simulink model "SmartMeter"  (R2023b)
settings: Solver=VariableStepAuto  StartTime=0.0  StopTime=3600*7.5  RelTol=1e-3
InitFcn:
  | Ts = 1; % Step time as 1second
StopFcn:
  | plotResults = true ;% turn off if unwanted
  | 
  | if plotResults
  | 
  | out = out_SmartMeterModel.SmartMeterValidationScope;
  | 
  | % Get Signals from simulation output.
  | time = out.time;
  | TestSignal = out.signals.values(:,1);
  | E_meas_15min = out.signals.values(:,2:3);
  | E_meas_hourly = out.signals.values(:,4:5);
  | price = out.signals.values(:,6:7);
  | Bill_hourly = out.signals.values(:,8:9);
  | 
  | %% Create Figure
  | fig_SmartMeterValidation_Results = figure;
  | 
  | % X-axis
  | step = 3600;
  | myxtick = 0:step:time(end);
  | myxticklabel = 0:time(end)/step ;
  | 
  | % TestSignal
  | subplot(5,1,1);
  | hold on;
  | plot(time, TestSignal, '-', 'LineWidth', 2,'Color','black');
  | ylim 'padded'
  | ylabel('Power (kW)');
  | xticks(myxtick);
  | xticklabels(myxticklabel);
  | xlim 'tight'
  | xlabel('Time (hours)');
  | title('Power');
  | grid on;
  | box on
  | 
  | % E 15
  | subplot(5,1,2);
  | hold on
  | stairs(time, E_meas_15min(:,1), 'LineWidth', 2);
  | stairs(time, E_meas_15min(:,2), 'LineWidth', 2);
  | ylim 'padded'
  | yticks(-1:0.25:1)
  | ylabel('Energy (kWh)');
  | xticks(myxtick);
  | xticklabels(myxticklabel);
  | xlim 'tight'
  | xlabel('Time (hours)');
  | %legend('BattPower','Location', 'northwest')
  | title('Measurements 15 min interval');
  | grid on;
  | box on
  | 
  | % E hourly
  | subplot(5,1,3);
  | hold on
  | stairs(time, E_meas_hourly(:,1), 'LineWidth', 2);
  | stairs(time, E_meas_hourly(:,2), 'LineWidth', 2);
  | ylim 'padded'
  | yticks(0:0.5:2)
  | ylabel('Energy (kWh)');
  | xticks(myxtick);
  | xticklabels(myxticklabel);
  | xlabel('Time (hours)');
  | xlim 'tight'
  | %legend('BattPower','Location', 'northwest')
  | title('Measurements hourly');
  | grid on;
  | box on
  | 
  | % price
  | subplot(5,1,4);
  | hold on
  | plot(time, price(:,1),':', 'LineWidth', 2,'Color','black')
  | plot(time, price(:,2),'-', 'LineWidth', 2,'Color','black')
  | ylim 'padded'
  | ylabel('DKK per kWh','Color','black');
  | xticks(myxtick);
  | xticklabels(myxticklabel);
  | xlim 'tight'
  | xlabel('Time (hours)');
  | legend( 'price','price shifted','Location', 'northeast');%, 'Location', 'northeast', 'Orientation', 'vertical', 'Position', [0.75, 0.2, 0.05, 0.05]);
  | title('Electricity spot price');
  | grid on;
  | box on
  | 
  | 
  | % Bill_hourly
  | subplot(5,1,5);
  | hold on
  | plot(time, Bill_hourly(:,1),'-', 'LineWidth', 2)
  | plot(time, Bill_hourly(:,2),'-', 'LineWidth', 2)
  | ylim 'padded'
  | ylabel('DKK');
  | xlim 'tight'
  | xticks(myxtick);
  | xticklabels(myxticklabel);
  | xlabel('Time (hours)');
  | %legend( 'price','price shifted','Location', 'northeast');
  | title('Hourly bill');
  | grid on;
  | box on
  | 
  | % Stretch Figure
  | figwidth = 8; % Width in inches
  | figheight = 6; % Height in inches
  | set(gcf, 'Units', 'Inches', 'Position', [1, 1, figwidth, figheight]);
  | 
  | % Save Files
  | saveas(fig_SmartMeterValidation_Results, 'SmartMeterValidation_Results', 'epsc')
  | saveas(fig_SmartMeterValidation_Results, 'SmartMeterValidation_Results', 'pdf')
  | 
  | disp('Figures saved as PDF and eps')
  | 
  | 
  | 
  | 
  | 
  | end
undefined symbols (not defined in the file): DiscIntNeverNeededParam, sigbuilder_block
libraries: dspsigops x2, spspowerguiLib x1
settings Model: Creator=leons  LastModifiedBy=leons
settings DataIOCC: ReturnWorkspaceOutputsName=out_SmartMeterModel

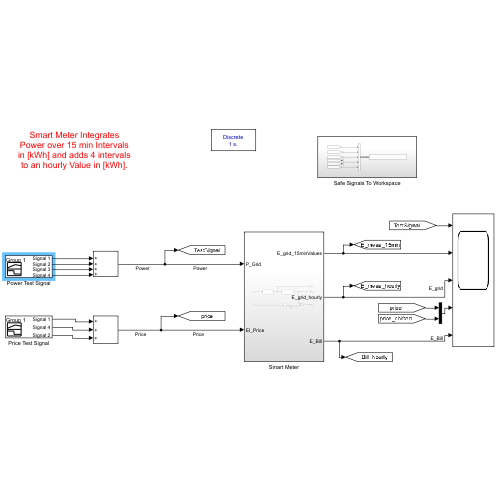
[thumbnail: Simulink's stored preview of the top-level diagram]
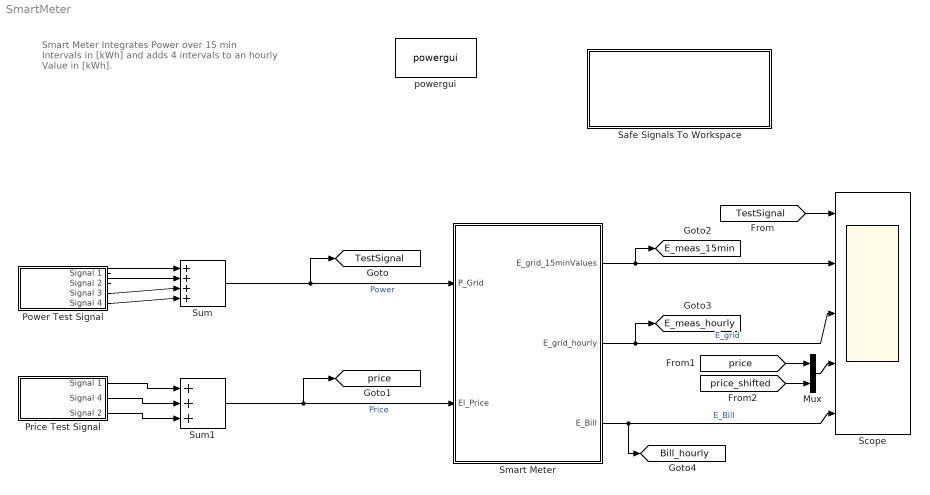
== system SmartMeter ==
  note: Smart Meter Integrates Power over 15 min Intervals in [kWh] and adds 4 intervals to an hourly Value in [kWh].
  Mux : Mux  Inputs=2
  Power Test Signal : Subsystem  Tag=STV Subsys  LoadFcn=sigbuilder_block('load');  StartFcn=sigbuilder_block('start');  StopFcn=sigbuilder_block('stop');  ClipboardFcn=sigbuilder_block('clipboard');  mask(Sigbuilder block){tuvar=[0:10]}
      mask help: Simulink:masks:SigbuilderBlock_MD
      mask init:
      | if ~strcmp(get_param(bdroot(gcbh),'SimulationStatus'),'stopped') tuvar = sigbuilder_block('maskInit'); end
      settings: CopyFcn=sigbuilder_block('copy');  DeleteFcn=sigbuilder_block('delete');  ModelCloseFcn=sigbuilder_block('modelClose');  PreSaveFcn=sigbuilder_block('preSave');  PauseFcn=sigbuilder_block('pause');  ContinueFcn=sigbuilder_block('continue');  NameChangeFcn=sigbuilder_block('namechange');  OpenFcn=sigbuilder_block('open',[38.4 99 759.6 460.8 ]);  CloseFcn=sigbuilder_block('close');
      mask Display: plot(0, 0, 100, 100,[2, 2, 32, 32, 2], [68, 8, 8, 68, 68],[32, 2], [38, 38], [32, 19, 2],[53, 60, 44], [32, 17, 17, 2],[16, 16, 31, 31]);txt = getActiveGroup(gcbh);text(2, 100, txt,'verticalAlignment', 'top');
  Price Test Signal : Subsystem  Tag=STV Subsys  LoadFcn=sigbuilder_block('load');  StartFcn=sigbuilder_block('start');  StopFcn=sigbuilder_block('stop');  ClipboardFcn=sigbuilder_block('clipboard');  mask(Sigbuilder block){tuvar=[0:10]}
      mask help: Simulink:masks:SigbuilderBlock_MD
      mask init:
      | if ~strcmp(get_param(bdroot(gcbh),'SimulationStatus'),'stopped') tuvar = sigbuilder_block('maskInit'); end
      settings: CopyFcn=sigbuilder_block('copy');  DeleteFcn=sigbuilder_block('delete');  ModelCloseFcn=sigbuilder_block('modelClose');  PreSaveFcn=sigbuilder_block('preSave');  PauseFcn=sigbuilder_block('pause');  ContinueFcn=sigbuilder_block('continue');  NameChangeFcn=sigbuilder_block('namechange');  OpenFcn=sigbuilder_block('open',[110.4 45 759.6 460.8 ]);  CloseFcn=sigbuilder_block('close');
      mask Display: plot(0, 0, 100, 100,[2, 2, 32, 32, 2], [68, 8, 8, 68, 68],[32, 2], [38, 38], [32, 19, 2],[53, 60, 44], [32, 17, 17, 2],[16, 16, 31, 31]);txt = getActiveGroup(gcbh);text(2, 100, txt,'verticalAlignment', 'top');
  Safe Signals To Workspace : Subsystem
  Scope : Scope  NumInputPorts=5
  Smart Meter : Subsystem
  Sum : Sum  Inputs=|++++
  Sum1 : Sum  Inputs=+++
  powergui : spspowerguiLib/powergui  Priority=1  SimulationMode=Discrete  SampleTime=Ts  frequency=60  Iterations=50  frequencyindice=60  Pbase=100e6  ErrMax=1e-4  UnitsV=kV  UnitsW=MW  buscounter=0  FunctionMessages=off  echomessages=off  EnableUseOfTLC=off  CurrentSourceSwitches=off  DisableSnubberDevices=off  DisableRonSwitches=off  DisableVfSwitches=off  DisplayEquations=off  AutomaticDiscreteSolvers=off  SolverType=Tustin/Backward Euler (TBE)  Interpol=off  ExternalGateDelay=off  methode=off  Ts=100  x0status=blocks  SPID=on  SwTol=0  HookPort=off  NonlinearTolerance=1e-4  nMaxIteration=100  ContinueOnMaxIteration=off  RestoreLinks=warning  ResistiveCurrentMeasurement=off  Frange=[0:2:500]  Ylog=off  Xlog=on  ShowGrid=off  save=off  variable=ZData  structure=0  ZoomFFT=off  StartTime=0.0  cycles=1  DisplayStyle=1  fundamental=60  FreqAxis=off  MaxFrequency=1000  frequencyindicesteady=1  RmsSteady=1  display=off
  tag scope: Bill_hourly=global, E_meas_15min=global, E_meas_hourly=global, TestSignal=global, price=global
  wires:
  Smart Meter/2(E_grid_hourly) -> [E_meas_hourly], Scope/3  "E_grid"
  Power Test Signal/4(Signal 4) -> Sum/4
  Power Test Signal/2(Signal 2) -> Sum/2
  Power Test Signal/1(Signal 1) -> Sum/1
  Power Test Signal/3(Signal 3) -> Sum/3
  Price Test Signal/1(Signal 1) -> Sum1/1
  Price Test Signal/2(Signal 4) -> Sum1/2
  Sum1/1 -> Smart Meter/2(El_Price), [price]  "Price"
  Smart Meter/3(E_Bill) -> Scope/5, [Bill_hourly]  "E_Bill"
  [TestSignal] -> Scope/1
  [price] -> Mux/1
  Sum/1 -> [TestSignal], Smart Meter/1(P_Grid)  "Power"
  Smart Meter/1(E_grid_15minValues) -> [E_meas_15min], Scope/2
  Mux/1 -> Scope/4
  [price_shifted] -> Mux/2
  Price Test Signal/3(Signal 2) -> Sum1/3

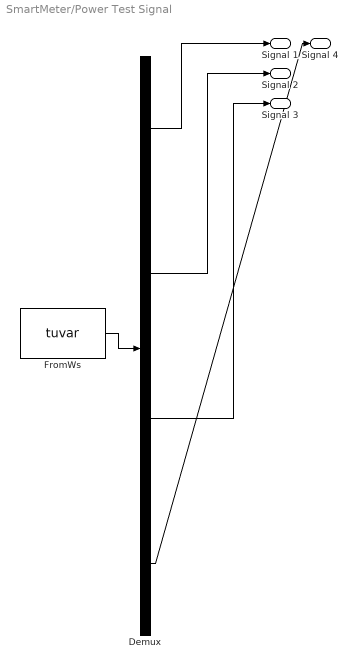
== system SmartMeter/Power Test Signal ==
  Demux : Demux  Tag=STV Demux
      settings: DisplayOption=none
  FromWs : FromWorkspace  Tag=STV FromWs  VariableName=tuvar
      SigBuilderData=|
      | common.afterFinalStr = 'Extrapolate'
      | common.sampleTime = 0
      | dataSet.timeRange = [0 25200]
      | dataSet.name = 'Group 1'
      | sbobj.Groups.Name = 'Group 1'
      | sbobj.Groups.Signals(1).Name = 'Signal 1'
      | sbobj.Groups.Signals(1).XData = [0 1 1 3600 3600 25200]
      | sbobj.Groups.Signals(1).YData = [0 0 1 1 0 0]
      | sbobj.Groups.Signals(2).Name = 'Signal 2'
      | sbobj.Groups.Signals(2).XData = [0 3600 3600 12600 12600 25200]
      | sbobj.Groups.Signals(2).YData = [0 0 2 2 0 0]
      | sbobj.Groups.Signals(3).Name = 'Signal 3'
      | sbobj.Groups.Signals(3).XData = [0 14402 14402 15298 15298 25200]
      | sbobj.Groups.Signals(3).YData = [0 0 2 -2 0 0]
      | sbobj.Groups.Signals(4).Name = 'Signal 4'
      | sbobj.Groups.Signals(4).XData = [0 18000 18000 19800 19800 25200]
      | sbobj.Groups.Signals(4).YData = [0 0 2 -2 0 0]
      | sbobj.Groups.TimeRange = [0 25200]
  Signal 1 : Outport  Tag=STV Outport
  Signal 2 : Outport  Tag=STV Outport  Port=2
  Signal 3 : Outport  Tag=STV Outport  Port=3
  Signal 4 : Outport  Tag=STV Outport  Port=4
  wires:
  Demux/3 -> Signal 3/1
  Demux/2 -> Signal 2/1
  FromWs/1 -> Demux/1
  Demux/1 -> Signal 1/1
  Demux/4 -> Signal 4/1

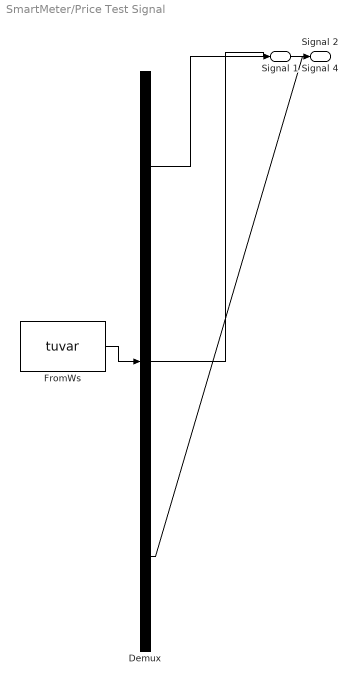
== system SmartMeter/Price Test Signal ==
  Demux : Demux  Tag=STV Demux  Outputs=3
      settings: DisplayOption=none
  FromWs : FromWorkspace  Tag=STV FromWs  VariableName=tuvar
      SigBuilderData=|
      | common.afterFinalStr = 'Extrapolate'
      | common.sampleTime = 0
      | dataSet.timeRange = [0 25200]
      | dataSet.name = 'Group 1'
      | sbobj.Groups.Name = 'Group 1'
      | sbobj.Groups.Signals(1).Name = 'Signal 1'
      | sbobj.Groups.Signals(1).XData = [0 1 1 3600 3600 25200]
      | sbobj.Groups.Signals(1).YData = [0 0 2 2 0 0]
      | sbobj.Groups.Signals(2).Name = 'Signal 4'
      | sbobj.Groups.Signals(2).XData = [0 7200 7200 25200]
      | sbobj.Groups.Signals(2).YData = [0 0 1 1]
      | sbobj.Groups.Signals(3).Name = 'Signal 2'
      | sbobj.Groups.Signals(3).XData = [0 3600 3600 7200 7200 25200]
      | sbobj.Groups.Signals(3).YData = [0 0 3 3 0 0]
      | sbobj.Groups.TimeRange = [0 25200]
  Signal 1 : Outport  Tag=STV Outport
  Signal 4 : Outport  Tag=STV Outport  Port=2
  Signal 2 : Outport  Tag=STV Outport  Port=3
  wires:
  FromWs/1 -> Demux/1
  Demux/1 -> Signal 1/1
  Demux/2 -> Signal 4/1
  Demux/3 -> Signal 2/1

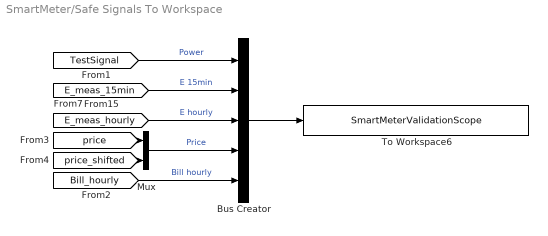
== system SmartMeter/Safe Signals To Workspace ==
  Bus Creator : BusCreator  Inputs=5
  Mux : Mux  Inputs=2
  To Workspace6 : ToWorkspace  VariableName=SmartMeterValidationScope  SaveFormat=Structure With Time  SampleTime=-1
  wires:
  Bus Creator/1 -> To Workspace6/1
  [E_meas_15min] -> Bus Creator/2  "E 15min"
  [TestSignal] -> Bus Creator/1  "Power"
  [E_meas_hourly] -> Bus Creator/3  "E hourly"
  Mux/1 -> Bus Creator/4  "Price"
  [Bill_hourly] -> Bus Creator/5  "Bill hourly"
  [price_shifted] -> Mux/2
  [price] -> Mux/1

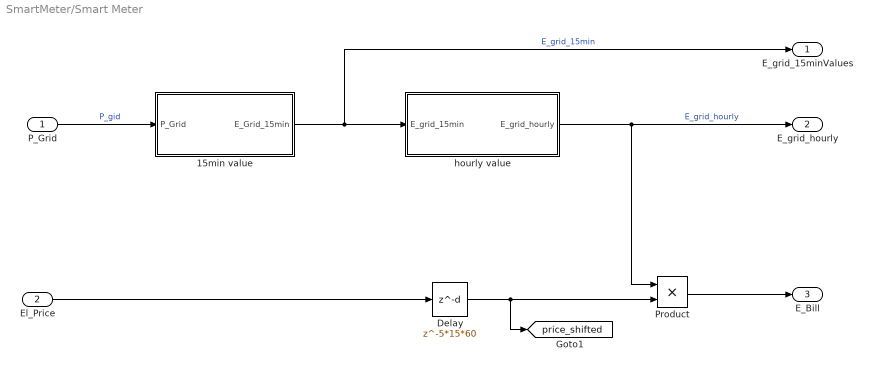
== system SmartMeter/Smart Meter ==
  P_Grid : Inport
  El_Price : Inport  Port=2
  15min value : Subsystem
  Delay : Delay  DelayLength=5*15*60  SampleTime=1
  Product : Product
  hourly value : Subsystem
  E_grid_15minValues : Outport
  E_grid_hourly : Outport  Port=2
  E_Bill : Outport  Port=3
  tag scope: price_shifted=global
  wires:
  P_Grid/1 -> 15min value/1(P_Grid)  "P_gid"
  15min value/1(E_Grid_15min) -> E_grid_15minValues/1, hourly value/1(E_grid_15min)  "E_grid_15min"
  hourly value/1("E_grid_hourly ") -> E_grid_hourly/1, Product/1  "E_grid_hourly"
  El_Price/1 -> Delay/1
  Delay/1 -> [price_shifted], Product/2
  Product/1 -> E_Bill/1

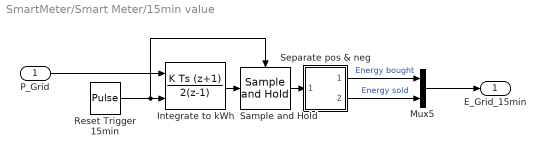
== system SmartMeter/Smart Meter/15min value ==
  P_Grid : Inport
  Integrate to kWh : DiscreteIntegrator  IntegratorMethod=Integration: Trapezoidal  gainval=1/(3600)  ExternalReset=falling  SampleTime=-1  ICPrevOutput=DiscIntNeverNeededParam  ICPrevScaledInput=DiscIntNeverNeededParam
  Mux5 : Mux  Inputs=2
  Reset Trigger 15min : DiscretePulseGenerator  Period=15*60  SampleTime=Ts
  Sample and Hold : dspsigops/Sample and Hold  trig=Rising edge  initCond=0  latchinput=off
  Separate pos & neg : Subsystem
  E_Grid_15min : Outport
  wires:
  Integrate to kWh/1 -> Sample and Hold/1
  Mux5/1 -> E_Grid_15min/1
  Sample and Hold/1 -> Separate pos & neg/1(Sig)
  Reset Trigger 15min/1 -> Integrate to kWh/2, Sample and Hold/Trigger
  Separate pos & neg/2(Neg) -> Mux5/2  "Energy sold"
  Separate pos & neg/1(Pos) -> Mux5/1  "Energy bought"
  P_Grid/1 -> Integrate to kWh/1

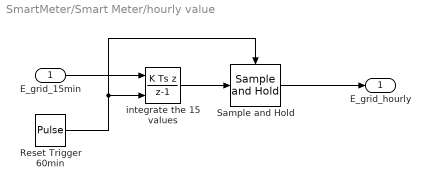
== system SmartMeter/Smart Meter/hourly value ==
  E_grid_15min : Inport
  Reset Trigger 60min : DiscretePulseGenerator  Period=60*60  PhaseDelay=900
  Sample and Hold : dspsigops/Sample and Hold  trig=Rising edge  initCond=0  latchinput=off
  integrate the 15 values : DiscreteIntegrator  IntegratorMethod=Integration: Backward Euler  gainval=1/(3600/4)  ExternalReset=falling  SampleTime=-1  ICPrevOutput=DiscIntNeverNeededParam  ICPrevScaledInput=DiscIntNeverNeededParam
  "E_grid_hourly " : Outport
  wires:
  Reset Trigger 60min/1 -> Sample and Hold/Trigger, integrate the 15 values/2
  integrate the 15 values/1 -> Sample and Hold/1
  Sample and Hold/1 -> "E_grid_hourly "/1
  E_grid_15min/1 -> integrate the 15 values/1

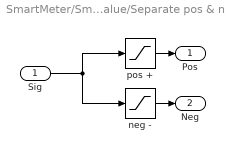
== system SmartMeter/Smart Meter/15min value/Separate pos & neg ==
  Sig : Inport
  neg - : Saturate  UpperLimit=0  LowerLimit=-inf
  pos + : Saturate  UpperLimit=inf  LowerLimit=0
  Pos : Outport
  Neg : Outport  Port=2
  wires:
  neg -/1 -> Neg/1
  pos +/1 -> Pos/1
  Sig/1 -> pos +/1, neg -/1
